simulink model "Missile_Plant_Trim_Analysis"  (R2021b)
settings: Solver=ode4  StartTime=0.0  StopTime=2  FixedStep=Step_Size  RelTol=1e-3
values from neighbouring files (symbols this model uses):
  D = 0.150    (= 0.15)    [Missile_Data.m]
  I_xx = 0.5 * Mass * ( D / 2 )^2    (= 0.084375)    [Missile_Data.m]
  I_yy = Mass * ( ( 1 / 12 ) * l^2 + ( 1 / 4 ) * ( D / 2 )^2 )    (= 6.5869975)    [Missile_Data.m]
  I_zz = I_yy    (= 6.5869975)    [Missile_Data.m]
  Mass = 30.0    (= 30)    [Missile_Data.m]
  S = ( pi / 4 ) * D^2    (= 0.0176714586764)    [Missile_Data.m]
  Tbl_CL_ALPHAT = [ -0.0988   -0.4859   -0.5870   -0.4802   -0.3334   -0.0210 ]    [Missile_Data.m]
  Tbl_CL_DEL_R = [ 5.2712    5.7640    6.1650    6.6234    7.1963    8.4110 ]    [Missile_Data.m]
  Tbl_CL_P = [ -17.9516  -19.6297  -20.9956  -22.5566  -24.5079  -28.6446 ]    [Missile_Data.m]
  Tbl_CM_0 = [ 0   -2.2250   -3.9280   -4.8580   -5.6940 ... (first row only)    [Missile_Data.m]
  Tbl_CM_DEL_P = [ -20.7182  -22.5631  -23.6059  -24.7632  -26.1269  -29.5646 ]    [Missile_Data.m]
  Tbl_CM_PHIT = [ 0   -0.0024   -0.0898   -0.2360   -0.3546 ... (first row only)    [Missile_Data.m]
  Tbl_CM_Q = [ -82.9643  -47.4409  -32.7732  -16.7304  -43.2010  -56.1499 ]    [Missile_Data.m]
  Tbl_CN_DEL_Y = [ -0.3616   -0.3938   -0.4120   -0.4322   -0.4560   -0.5160 ]    [Missile_Data.m]
  Tbl_CN_PHIT = [ 0    0.0040    0.0098    0.1116    0.3049 ... (first row only)    [Missile_Data.m]
  Tbl_CN_R = [ -82.9643  -47.4409  -32.7732  -16.7304  -43.2010  -56.1499 ]    [Missile_Data.m]
  Tbl_CX_0 = [ -0.3840   -0.3670   -0.3550   -0.3460   -0.3390   -0.3410 ]    [Missile_Data.m]
  Tbl_CX_ALPHAT = [ 0.0788    0.0752    0.0680    0.0573    0.0573    0.0573 ]    [Missile_Data.m]
  Tbl_CX_DEL_EFF = [ -16.8080  -17.8585  -18.9090  -19.9595  -20.4847  -23.1110 ]    [Missile_Data.m]
  Tbl_CY_DEL_Y = [ 5.3056    5.7754    6.0504    6.3484    6.6921    7.5745 ]    [Missile_Data.m]
  Tbl_CY_PHIT = [ 0    0.0070    0.0819    0.2313    0.2992 ... (first row only)    [Missile_Data.m]
  Tbl_CZ_0 = [ 0   -2.0680   -3.9700   -5.4250   -6.6810 ... (first row only)    [Missile_Data.m]
  Tbl_CZ_DEL_P = [ -5.3056   -5.7754   -6.0504   -6.3484   -6.6921   -7.5745 ]    [Missile_Data.m]
  Tbl_CZ_PHIT = [ 0    0.0089    0.1842    0.3041    0.2039 ... (first row only)    [Missile_Data.m]
  UNIT_GRAV = 9.81    [Sim_Parameters.m]
  windOn = 0    [Sim_Parameters.m]
  XCG = 0.809    [Missile_Data.m]
  XREF = 0.809    [Missile_Data.m]
undefined symbols (not defined in the file or in its folder): F, Light, MIL
libraries: aerolibwind2 x3, aerolibasang x3, sharedtransform x2, aerolibatmos2 x1, shared6dof x1, aerolibnav x1, sharedutil x1, simulink_extras x1
settings Model: Creator=Tiga  LastModifiedBy=Tiga
settings DataIOCC: SaveOutput=off  SaveTime=off

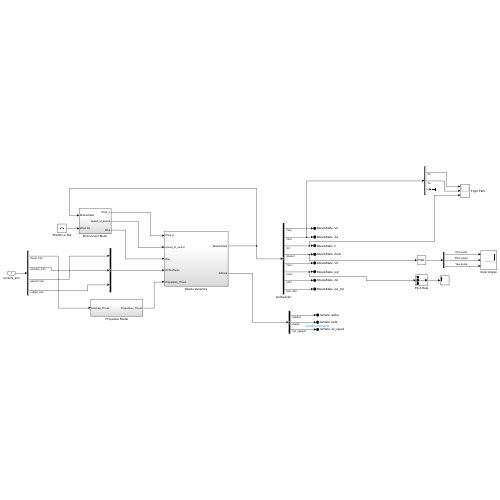
[thumbnail: Simulink's stored preview of the top-level diagram]
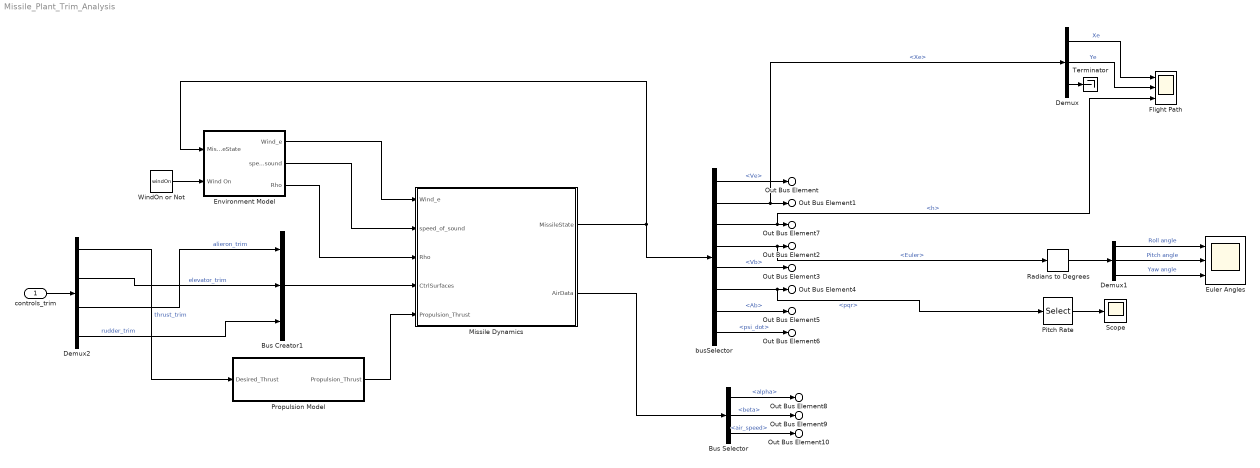
== system Missile_Plant_Trim_Analysis ==
  controls_trim : Inport
  Bus Creator1 : BusCreator  Inputs=3
  Bus Selector : BusSelector  OutputSignals=alpha,beta,air_speed
  Demux : Demux  Outputs=3
  Demux1 : Demux  Outputs=3
  Demux2 : Demux
  Environment Model : Subsystem
  Euler Angles : Scope  NumInputPorts=3
  Flight Path : Scope  NumInputPorts=3
  Missile Dynamics : Subsystem
  Pitch Rate : Selector  InputPortWidth=3  IndexOptions=Index vector (dialog)  Indices=[2]  OutputSizes=1
  Propulsion Model : Subsystem
  Radians to Degrees : simulink_extras/Transformations/Radians to Degrees
  Scope : Scope
  Terminator : Terminator
  WindOn or Not : Constant  Value=windOn
  busSelector : BusSelector  OutputSignals=Ve,Xe,h,Euler,Vb,pqr,Ab,psi_dot
  Out Bus Element : Outport  PortName=MissileState  Element=Ve
  Out Bus Element1 : Outport  PortName=MissileState  Element=Xe
  Out Bus Element2 : Outport  PortName=MissileState  Element=Euler
  Out Bus Element3 : Outport  PortName=MissileState  Element=Vb
  Out Bus Element4 : Outport  PortName=MissileState  Element=pqr
  Out Bus Element5 : Outport  PortName=MissileState  Element=Ab
  Out Bus Element6 : Outport  PortName=MissileState  Element=psi_dot
  Out Bus Element7 : Outport  PortName=MissileState  Element=h
  Out Bus Element8 : Outport  Port=2  PortName=AirData  Element=alpha
  Out Bus Element9 : Outport  Port=2  PortName=AirData  Element=beta
  Out Bus Element10 : Outport  Port=2  PortName=AirData  Element=air_speed
  wires:
  busSelector/8 -> Out Bus Element6/1  "<psi_dot>"
  busSelector/7 -> Out Bus Element5/1  "<Ab>"
  busSelector/6 -> Pitch Rate/1, Out Bus Element4/1  "<pqr>"
  busSelector/5 -> Out Bus Element3/1  "<Vb>"
  busSelector/4 -> Radians to Degrees/1, Out Bus Element2/1  "<Euler>"
  busSelector/2 -> Out Bus Element1/1, Demux/1  "<Xe>"
  busSelector/1 -> Out Bus Element/1  "<Ve>"
  Missile Dynamics/1(MissileState) -> busSelector/1, Environment Model/1(MissileState)
  Environment Model/3(Rho) -> Missile Dynamics/3(Rho)
  WindOn or Not/1 -> Environment Model/2(Wind On)
  Environment Model/1(Wind_e) -> Missile Dynamics/1(Wind_e)
  Propulsion Model/1(Propulsion_Thrust) -> Missile Dynamics/5(Propulsion_Thrust)
  Environment Model/2(speed_of_sound) -> Missile Dynamics/2(speed_of_sound)
  busSelector/3 -> Flight Path/3, Out Bus Element7/1  "<h>"
  Radians to Degrees/1 -> Demux1/1
  Demux1/2 -> Euler Angles/2  "Pitch angle"
  Demux1/3 -> Euler Angles/3  "Yaw angle"
  Demux1/1 -> Euler Angles/1  "Roll angle"
  Pitch Rate/1 -> Scope/1
  Demux/1 -> Flight Path/1  "Xe"
  Demux/2 -> Flight Path/2  "Ye"
  Demux/3 -> Terminator/1
  controls_trim/1 -> Demux2/1
  Demux2/1 -> Propulsion Model/1(Desired_Thrust)  "thrust_trim"
  Demux2/3 -> Bus Creator1/1  "alieron_trim"
  Demux2/2 -> Bus Creator1/2  "elevator_trim"
  Demux2/4 -> Bus Creator1/3  "rudder_trim"
  Bus Creator1/1 -> Missile Dynamics/4(CtrlSurfaces)
  Missile Dynamics/2(AirData) -> Bus Selector/1
  Bus Selector/1 -> Out Bus Element8/1  "<alpha>"
  Bus Selector/2 -> Out Bus Element9/1  "<beta>"
  Bus Selector/3 -> Out Bus Element10/1  "<air_speed>"

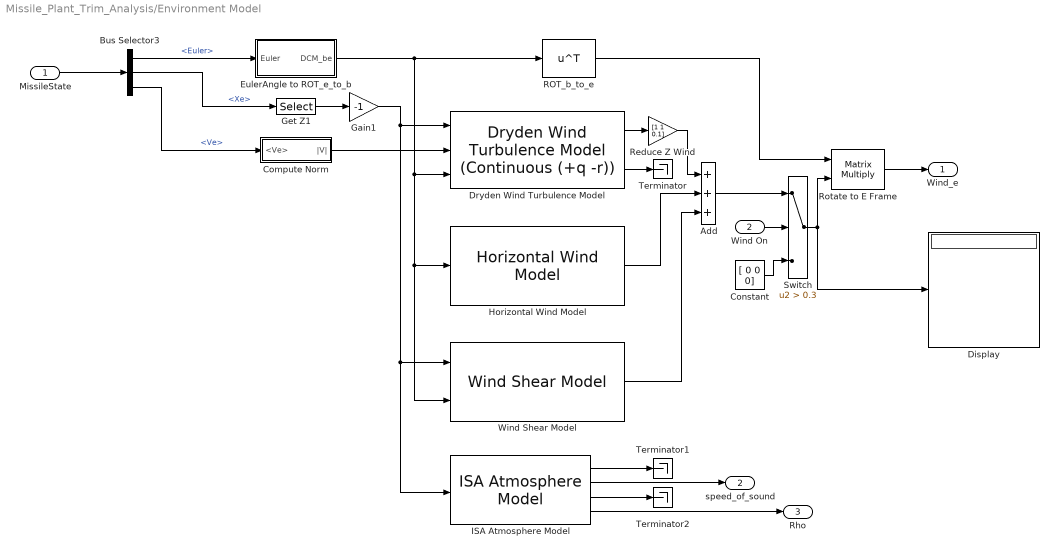
== system Missile_Plant_Trim_Analysis/Environment Model ==
  MissileState : Inport
  Wind On : Inport  Port=2
  Add : Sum  Inputs=3
  Bus Selector3 : BusSelector  OutputSignals=Euler,Xe,Ve
  Compute Norm : Subsystem
  Constant : Constant  Value=[ 0 0 0]
      settings: AttributesFormatString=%<Value>
  Display : Display
  Dryden Wind Turbulence Model : aerolibwind2/Dryden Wind Turbulence Model  (Continuous (+q -r))  units=Metric (MKS)  spec=MIL-F-8785C  model=Continuous Dryden (+q -r)  W20=12  Wdeg=180  TurbProb=10^-2 - Light  L_high=533.4  Wingspan=l  ts=0.01  Seed=[23341 23342 23343 23344]  T_on=on
  EulerAngle to ROT_e_to_b : Subsystem
  Gain1 : Gain  Gain=-1
      settings: AttributesFormatString=Z to Alt
  Get Z1 : Selector  InputPortWidth=3  IndexOptions=Index vector (dialog)  Indices=[3]  OutputSizes=[(-2)]
  "Horizontal Wind Model " : aerolibwind2/Horizontal Wind Model  units=Metric (MKS)  Vw_source=Internal  Vwind=12  W_source=Internal  Wdeg=90
      settings: SourceProductBaseCode=AE
  ISA Atmosphere Model : aerolibatmos2/ISA Atmosphere Model  custom=off  g=9.80665  gamma=1.4  R=287.0531  L=0.0065  h_trop=11000  h_strat=20000  rho0=1.225  P0=101325  T0=288.15  h0=0
  ROT_b_to_e : Math  Operator=transpose  SignedPower=on  SaturateOnIntegerOverflow=on
  Reduce Z Wind : Gain  Gain=[1 1 0.1]
      settings: AttributesFormatString=%<Gain>
  Rotate to E Frame : Product  Multiplication=Matrix(*)
  Switch : Switch  Criteria=u2 > Threshold  Threshold=0.3
  Terminator : Terminator
  Terminator1 : Terminator
  Terminator2 : Terminator
  Wind Shear Model : aerolibwind2/Wind Shear Model  units=Metric (MKS)  phase=Category C - Terminal Flight Phase  W_20=15  Wdeg=0
  Wind_e : Outport  Unit=m/s  VectorParamsAs1DForOutWhenUnconnected=off
  speed_of_sound : Outport  Port=2  Unit=m/s  VectorParamsAs1DForOutWhenUnconnected=off
  Rho : Outport  Port=3  Unit=kg/m^3  VectorParamsAs1DForOutWhenUnconnected=off
  wires:
  Compute Norm/1(|V|) -> Dryden Wind Turbulence Model/2
  Bus Selector3/3 -> Compute Norm/1(<Ve>)  "<Ve>"
  EulerAngle to ROT_e_to_b/1(DCM_be) -> ROT_b_to_e/1, Dryden Wind Turbulence Model/3, "Horizontal Wind Model "/1, Wind Shear Model/2
  Bus Selector3/1 -> EulerAngle to ROT_e_to_b/1(Euler)  "<Euler>"
  ISA Atmosphere Model/3 -> Terminator2/1
  ISA Atmosphere Model/1 -> Terminator1/1
  ISA Atmosphere Model/2 -> speed_of_sound/1
  ISA Atmosphere Model/4 -> Rho/1
  Wind Shear Model/1 -> Add/3
  Wind On/1 -> Switch/2
  Add/1 -> Switch/1
  Reduce Z Wind/1 -> Add/1
  "Horizontal Wind Model "/1 -> Add/2
  Gain1/1 -> Dryden Wind Turbulence Model/1, Wind Shear Model/1, ISA Atmosphere Model/1
  MissileState/1 -> Bus Selector3/1
  Dryden Wind Turbulence Model/1 -> Reduce Z Wind/1
  Switch/1 -> Display/1, Rotate to E Frame/2
  Rotate to E Frame/1 -> Wind_e/1
  ROT_b_to_e/1 -> Rotate to E Frame/1
  Get Z1/1 -> Gain1/1
  Constant/1 -> Switch/3
  Dryden Wind Turbulence Model/2 -> Terminator/1
  Bus Selector3/2 -> Get Z1/1  "<Xe>"

== system Missile_Plant_Trim_Analysis/Missile Dynamics ==
  Wind_e : Inport
  speed_of_sound : Inport  Port=2
  Rho : Inport  Port=3
  CtrlSurfaces : Inport  Port=4
  Propulsion_Thrust : Inport  Port=5
  6DOF Nonlinear Equations of Motion : Subsystem
  Aerodynamic Forces and Moments : Subsystem
  Total Force and Moment : Subsystem
  MissileState : Outport
  AirData : Outport  Port=2
  wires:
  CtrlSurfaces/1 -> Aerodynamic Forces and Moments/5(CtrlSurfaces)
  Rho/1 -> Aerodynamic Forces and Moments/4(Rho)
  speed_of_sound/1 -> Aerodynamic Forces and Moments/3(speed_of_sound)
  Wind_e/1 -> Aerodynamic Forces and Moments/1(Wind_e)
  6DOF Nonlinear Equations of Motion/1(MissileState) -> Aerodynamic Forces and Moments/2(MissileState), MissileState/1, Total Force and Moment/3(MissileState)
  Propulsion_Thrust/1 -> Total Force and Moment/2(Propulsion_Thrust)
  Aerodynamic Forces and Moments/1(Fm_b) -> Total Force and Moment/1(Aero-Force-Moment)
  Total Force and Moment/1(Total_Force_Moment) -> 6DOF Nonlinear Equations of Motion/1(FM_b)
  Aerodynamic Forces and Moments/2(AirData) -> AirData/1

== system Missile_Plant_Trim_Analysis/Propulsion Model ==
  note: F_Tx
  Desired_Thrust : Inport
  F_Ty : Constant  Value=0
  F_Tz : Constant  Value=0
  L_T : Constant  Value=0
  M_T : Constant  Value=0
  Mux : Mux  Inputs=3
  Mux1 : Mux  Inputs=3
  Mux2 : Mux  Inputs=2
  N_T : Constant  Value=0
  Propulsion_Thrust : Outport
  wires:
  N_T/1 -> Mux1/3
  M_T/1 -> Mux1/2
  L_T/1 -> Mux1/1
  F_Tz/1 -> Mux/3
  F_Ty/1 -> Mux/2
  Desired_Thrust/1 -> Mux/1
  Mux2/1 -> Propulsion_Thrust/1
  Mux1/1 -> Mux2/2
  Mux/1 -> Mux2/1

== system Missile_Plant_Trim_Analysis/Environment Model/Compute Norm ==
  <Ve> : Inport
  Dot Product : DotProduct  InputSameDT=on  OutDataTypeStr=Inherit: Inherit via internal rule
  Sqrt : Sqrt  SaturateOnIntegerOverflow=on
  Zero Bound : Saturate  UpperLimit=inf  LowerLimit=0.001
      settings: AttributesFormatString="[%<LowerLimit>  %<UpperLimit>]"
  |V| : Outport
  wires:
  Zero Bound/1 -> Sqrt/1
  Dot Product/1 -> Zero Bound/1
  Sqrt/1 -> |V|/1
  <Ve>/1 -> Dot Product/1, Dot Product/2

== system Missile_Plant_Trim_Analysis/Environment Model/EulerAngle to ROT_e_to_b ==
  Euler : Inport
  Rotation Angles to Direction Cosine Matrix : sharedtransform/Rotation Angles to Direction Cosine Matrix  rotationOrder=ZYX  aMode=aMode
      settings: SourceProductBaseCode=AE,PW,DR,MT,UV,VE
  Selector : Selector  InputPortWidth=3  IndexOptions=Index vector (dialog)  Indices=[3 2 1]  OutputSizes=1
  DCM_be : Outport
  wires:
  Euler/1 -> Selector/1
  Selector/1 -> Rotation Angles to Direction Cosine Matrix/1  "3 (rad)"
  Rotation Angles to Direction Cosine Matrix/1 -> DCM_be/1

== system Missile_Plant_Trim_Analysis/Missile Dynamics/6DOF Nonlinear Equations of Motion ==
  FM_b : Inport
  6DOF (Euler Angles) : shared6dof/6DOF (Euler Angles)  units=Metric (MKS)  mtype=Fixed  rep=Euler Angles  xme_0=Init_Pos  Vm_0=Init_Vel  eul_0=[ 0.0, 0.0, 0.0 ]  pm_0=Init_Rate  mass_0=Mass  mass_e=0.5  mass_f=2.0  inertia=eye(3).*[I_xx;I_yy;I_zz]  inertia_e=eye(3)  inertia_f=2*eye(3)  k_quat=1.0  vre_flag=on  abi_flag=off  aMode=aMode  xme_statename=''  Vm_statename=''  eul_statename=''  quat_statename=''  pm_statename=''  mass_statename=''
      settings: SourceProductBaseCode=AE
  Bus Creator : BusCreator  Inputs=9
  Compute psi_dot : Subsystem
  Constant : Constant  Value=[0 0 0]
      settings: AttributesFormatString=%<Value>
  Demux2 : Demux  Outputs=2
  Three-axis Accelerometer : aerolibnav/Three-axis Accelerometer  units=Metric (MKS)  acc=[0 0 0]  gtype=off  dtype_a=off  w_a=190  z_a=0.707  a_sf_cc=[1 0 0; 0 1 0; 0 0 1]  a_bias=[0 0 0]  a_Ts=0  a_rand=off  a_seeds=[23093 23094 23095]  a_pow=[0.001 0.001 0.001]  a_sat="[-inf  -inf  -inf  inf inf inf]"
      settings: SourceProductBaseCode=AE
  Z_to_Altitude : Subsystem
  MissileState : Outport
  wires:
  Bus Creator/1 -> MissileState/1
  Three-axis Accelerometer/1 -> Bus Creator/8  "Ab"
  6DOF (Euler Angles)/2 -> Z_to_Altitude/1(Xe), Bus Creator/2  "Xe"
  Demux2/1 -> 6DOF (Euler Angles)/1
  6DOF (Euler Angles)/6 -> Three-axis Accelerometer/2, Bus Creator/7, Compute psi_dot/2(G)  "pqr"
  Demux2/2 -> 6DOF (Euler Angles)/2
  6DOF (Euler Angles)/1 -> Bus Creator/1  "Ve"
  6DOF (Euler Angles)/7 -> Three-axis Accelerometer/3
  6DOF (Euler Angles)/5 -> Bus Creator/6  "Vb"
  Constant/1 -> Three-axis Accelerometer/4
  6DOF (Euler Angles)/3 -> Compute psi_dot/1(Euler), Bus Creator/4  "Euler"
  FM_b/1 -> Demux2/1
  Compute psi_dot/1(psi_dot) -> Bus Creator/9  "psi_dot"
  6DOF (Euler Angles)/8 -> Three-axis Accelerometer/1
  6DOF (Euler Angles)/4 -> Bus Creator/5  "DCM_be"
  Z_to_Altitude/1(h) -> Bus Creator/3  "h"

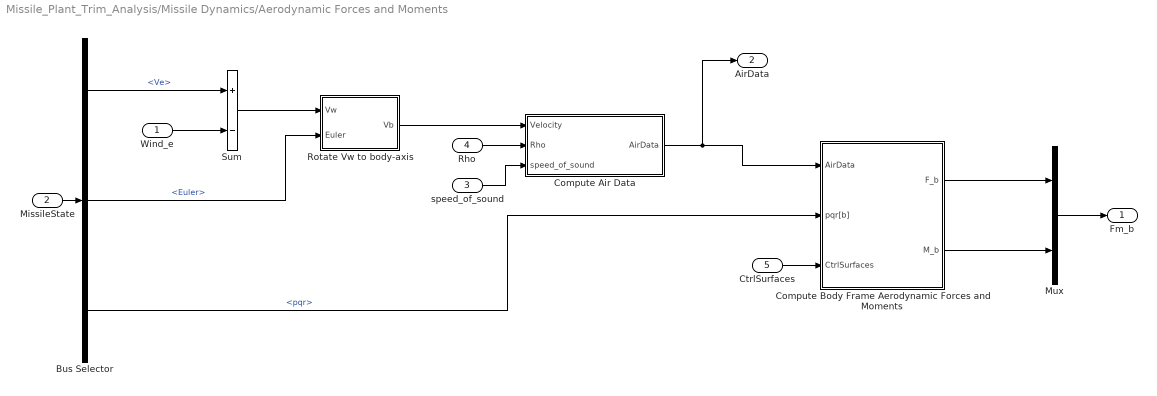
== system Missile_Plant_Trim_Analysis/Missile Dynamics/Aerodynamic Forces and Moments ==
  Wind_e : Inport
  MissileState : Inport  Port=2
  speed_of_sound : Inport  Port=3  Unit=m/s
  Rho : Inport  Port=4  Unit=kg/m^3
  CtrlSurfaces : Inport  Port=5
  Bus Selector : BusSelector  OutputSignals=Ve,Euler,pqr
  Compute Air Data : Subsystem
  Compute Body Frame Aerodynamic Forces and Moments : Subsystem
  Mux : Mux  Inputs=2
  Rotate Vw to body-axis : Subsystem
  Sum : Sum  Inputs=+-
  Fm_b : Outport
  AirData : Outport  Port=2
  wires:
  Compute Body Frame Aerodynamic Forces and Moments/1(F_b) -> Mux/1
  Compute Body Frame Aerodynamic Forces and Moments/2(M_b) -> Mux/2
  Mux/1 -> Fm_b/1
  CtrlSurfaces/1 -> Compute Body Frame Aerodynamic Forces and Moments/3(CtrlSurfaces)
  Compute Air Data/1(AirData) -> AirData/1, Compute Body Frame Aerodynamic Forces and Moments/1(AirData)
  speed_of_sound/1 -> Compute Air Data/3(speed_of_sound)
  Rho/1 -> Compute Air Data/2(Rho)
  Rotate Vw to body-axis/1(Vb) -> Compute Air Data/1(Velocity)
  Bus Selector/2 -> Rotate Vw to body-axis/2(Euler)  "<Euler>"
  Bus Selector/3 -> Compute Body Frame Aerodynamic Forces and Moments/2(pqr[b])  "<pqr>"
  MissileState/1 -> Bus Selector/1
  Wind_e/1 -> Sum/2
  Sum/1 -> Rotate Vw to body-axis/1(Vw)
  Bus Selector/1 -> Sum/1  "<Ve>"

== system Missile_Plant_Trim_Analysis/Missile Dynamics/Total Force and Moment ==
  Aero-Force-Moment : Inport
  Propulsion_Thrust : Inport  Port=2
  MissileState : Inport  Port=3
  Demux : Demux  Outputs=2
  Demux1 : Demux  Outputs=2
  Gravity : Subsystem
  Gravity's effect on moment : Constant  Value=0
  Mux : Mux  Inputs=2
  Total Force : Sum  Inputs=+++
  Total Moment : Sum  Inputs=+++
  Total_Force_Moment : Outport
  wires:
  Aero-Force-Moment/1 -> Demux/1
  Propulsion_Thrust/1 -> Demux1/1
  Demux/1 -> Total Force/1  "Aero-F"
  Demux1/1 -> Total Force/2  "Prop-F"
  MissileState/1 -> Gravity/1(MissileState)
  Gravity/1(Gravitational Force) -> Total Force/3  "Gravity-F"
  Demux/2 -> Total Moment/1  "Aero-M"
  Demux1/2 -> Total Moment/2  "Prop-M"
  Gravity's effect on moment/1 -> Total Moment/3
  Total Force/1 -> Mux/1
  Total Moment/1 -> Mux/2
  Mux/1 -> Total_Force_Moment/1

== system Missile_Plant_Trim_Analysis/Missile Dynamics/6DOF Nonlinear Equations of Motion/Compute psi_dot ==
  Euler : Inport
  G : Inport  Port=2
  Mux1 : Mux  Inputs=2
  psidot : Fcn  Expr=(u[5]*sin(u[1])+u[6]*cos(u[1]))/cos(u[2])
  psi_dot : Outport  Unit=rad/S  VectorParamsAs1DForOutWhenUnconnected=off
  wires:
  Euler/1 -> Mux1/1
  Mux1/1 -> psidot/1
  psidot/1 -> psi_dot/1  "psi_dot"
  G/1 -> Mux1/2

== system Missile_Plant_Trim_Analysis/Missile Dynamics/6DOF Nonlinear Equations of Motion/Z_to_Altitude ==
  Xe : Inport
  Gain : Gain  Gain=-1
  Selector : Selector  InputPortWidth=3  IndexOptions=Index vector (dialog)  Indices=[3]  OutputSizes=1
  h : Outport
  wires:
  Xe/1 -> Selector/1
  Selector/1 -> Gain/1
  Gain/1 -> h/1

== system Missile_Plant_Trim_Analysis/Missile Dynamics/Aerodynamic Forces and Moments/Compute Air Data ==
  Velocity : Inport
  Rho : Inport  Port=2  Unit=kg/m^3
  speed_of_sound : Inport  Port=3  Unit=m/s
  Bus Creator : BusCreator  Inputs=5
  Dynamic Pressure : aerolibasang/Dynamic Pressure
  "Incidence, Sideslip, & Airspeed" : aerolibasang/Incidence, Sideslip, & Airspeed
  Mach Number : aerolibasang/Mach Number
      settings: SourceProductBaseCode=AE
  AirData : Outport
  wires:
  "Incidence, Sideslip, & Airspeed"/3 -> Bus Creator/3  "air_speed"
  Bus Creator/1 -> AirData/1
  speed_of_sound/1 -> Mach Number/2
  "Incidence, Sideslip, & Airspeed"/2 -> Bus Creator/2  "beta"
  Dynamic Pressure/1 -> Bus Creator/4  "dynamic_pressure"
  "Incidence, Sideslip, & Airspeed"/1 -> Bus Creator/1  "alpha"
  Rho/1 -> Dynamic Pressure/2
  Mach Number/1 -> Bus Creator/5  "mach"
  Velocity/1 -> Dynamic Pressure/1, Mach Number/1, "Incidence, Sideslip, & Airspeed"/1

== system Missile_Plant_Trim_Analysis/Missile Dynamics/Aerodynamic Forces and Moments/Compute Body Frame Aerodynamic Forces and Moments ==
  AirData : Inport
  pqr[b] : Inport  Port=2
  CtrlSurfaces : Inport  Port=3
  Bus Selector : BusSelector  OutputSignals=dynamic_pressure
  Compute Aeroballistics Frame Aerodynamics Coefficients : Subsystem
  Compute Body Frame Aerodynamic Forces and Moments : Subsystem
  Convert AeroCoeffs_a to AeroCoeffs_b : Subsystem
  Display : Display
  F_b : Outport
  M_b : Outport  Port=2
  wires:
  Convert AeroCoeffs_a to AeroCoeffs_b/2(Aero-M-Coeffs_b) -> Compute Body Frame Aerodynamic Forces and Moments/3(Aero-M-Coeffs_b)
  Compute Aeroballistics Frame Aerodynamics Coefficients/2(Aero-M-Coeffs_a) -> Convert AeroCoeffs_a to AeroCoeffs_b/2(Aero-M-Coeffs_a)
  Compute Aeroballistics Frame Aerodynamics Coefficients/3(ROT_b_to_a) -> Convert AeroCoeffs_a to AeroCoeffs_b/3(ROT_b_to_a)
  Bus Selector/1 -> Compute Body Frame Aerodynamic Forces and Moments/1(dynamic_pressure)  "<dynamic_pressure>"
  Compute Body Frame Aerodynamic Forces and Moments/2(M_b) -> M_b/1
  Convert AeroCoeffs_a to AeroCoeffs_b/1(Aero-F-Coeffs_b) -> Compute Body Frame Aerodynamic Forces and Moments/2(Aero-F-Coeffs_b)
  Compute Body Frame Aerodynamic Forces and Moments/1(F_b) -> F_b/1
  Compute Aeroballistics Frame Aerodynamics Coefficients/1(Aero-F-Coeffs_a) -> Convert AeroCoeffs_a to AeroCoeffs_b/1(Aero-F-Coeffs_a)
  pqr[b]/1 -> Compute Aeroballistics Frame Aerodynamics Coefficients/2(pqr[b])
  CtrlSurfaces/1 -> Compute Aeroballistics Frame Aerodynamics Coefficients/3(CtrlSurfaces)
  AirData/1 -> Display/1, Compute Aeroballistics Frame Aerodynamics Coefficients/1(AirData), Bus Selector/1

== system Missile_Plant_Trim_Analysis/Missile Dynamics/Aerodynamic Forces and Moments/Rotate Vw to body-axis ==
  Vw : Inport
  Euler : Inport  Port=2
  EulerAngle to ROT_e_to_b : Subsystem
  RL2B * Vw : Product  Multiplication=Matrix(*)  InputSameDT=on  SaturateOnIntegerOverflow=on  OutDataTypeStr=Inherit: Same as first input
  Vb : Outport  Unit=m/s  VectorParamsAs1DForOutWhenUnconnected=off
  wires:
  EulerAngle to ROT_e_to_b/1(DCM_be) -> RL2B * Vw/1
  Euler/1 -> EulerAngle to ROT_e_to_b/1(Euler)
  Vw/1 -> RL2B * Vw/2
  RL2B * Vw/1 -> Vb/1

== system Missile_Plant_Trim_Analysis/Missile Dynamics/Total Force and Moment/Gravity ==
  MissileState : Inport
  Bus Selector : BusSelector  OutputSignals=DCM_be
  Constant : Constant  Value=Mass
  Constant1 : Constant  Value=0
  Matrix Multiply : Product  Multiplication=Matrix(*)
  Mux : Mux  Inputs=3
  UNIT_GRAV : Gain  Gain=UNIT_GRAV
  Gravitational Force : Outport
  wires:
  UNIT_GRAV/1 -> Mux/3
  Constant/1 -> UNIT_GRAV/1
  Constant1/1 -> Mux/2, Mux/1
  MissileState/1 -> Bus Selector/1
  Bus Selector/1 -> Matrix Multiply/1  "<DCM_be>"
  Mux/1 -> Matrix Multiply/2
  Matrix Multiply/1 -> Gravitational Force/1

== system Missile_Plant_Trim_Analysis/Missile Dynamics/Aerodynamic Forces and Moments/Compute Body Frame Aerodynamic Forces and Moments/Compute Aeroballistics Frame Aerodynamics Coefficients ==
  AirData : Inport
  pqr[b] : Inport  Port=2
  CtrlSurfaces : Inport  Port=3
  Calculate Coefficient Parameters : Subsystem
  Compute Aero-F-Coeffs_a : Subsystem
  Compute Aero-M-Coeffs_a : Subsystem
  Mach_Number Index Search : PreLookup  BreakpointsData=Tbl_MACH  OutputSelection=Index and fraction as bus  ExtrapMethod=Linear
  alpha_T Index Search : PreLookup  BreakpointsData=Tbl_ALPHAT  OutputSelection=Index and fraction as bus  BeginIndexSearchUsingPreviousIndexResult=on  ExtrapMethod=Linear
  Aero-F-Coeffs_a : Outport
  Aero-M-Coeffs_a : Outport  Port=2
  ROT_b_to_a : Outport  Port=3
  wires:
  Compute Aero-M-Coeffs_a/1(Aero-M-Coeffs_a) -> Aero-M-Coeffs_a/1
  Calculate Coefficient Parameters/9(pqr[a]) -> Compute Aero-M-Coeffs_a/8(pqr[a])
  Calculate Coefficient Parameters/8(geo_param) -> Compute Aero-M-Coeffs_a/7(geo_param)
  Calculate Coefficient Parameters/7(D/2V) -> Compute Aero-M-Coeffs_a/6(D/2V)
  Compute Aero-F-Coeffs_a/1(Aero-F-Coeffs_a) -> Aero-F-Coeffs_a/1, Compute Aero-M-Coeffs_a/9(Aero-F-Coeffs_a)
  Calculate Coefficient Parameters/6(roll_angle_T) -> Compute Aero-M-Coeffs_a/3(roll_angle_T), Compute Aero-F-Coeffs_a/4(roll_angle_T)
  Calculate Coefficient Parameters/5(CtrlSurfaces[a]) -> Compute Aero-M-Coeffs_a/5(CtrlSurfaces[a]), Compute Aero-F-Coeffs_a/6(CtrlSurfaces[a])
  Calculate Coefficient Parameters/4(dEFF) -> Compute Aero-F-Coeffs_a/5(dEFF)
  Mach_Number Index Search/1 -> Compute Aero-F-Coeffs_a/2(Mach_Number_index), Compute Aero-M-Coeffs_a/2(Mach_Number_index)
  alpha_T Index Search/1 -> Compute Aero-F-Coeffs_a/1(alpha_T_index), Compute Aero-M-Coeffs_a/1(alpha_T_index)
  Calculate Coefficient Parameters/3(Mach_Number) -> Mach_Number Index Search/1
  Calculate Coefficient Parameters/2(alpha_T) -> Compute Aero-F-Coeffs_a/3(alpha_T), Compute Aero-M-Coeffs_a/4(alpha_T), alpha_T Index Search/1
  Calculate Coefficient Parameters/1(ROT_b_to_a) -> ROT_b_to_a/1
  AirData/1 -> Calculate Coefficient Parameters/1(AirData)
  pqr[b]/1 -> Calculate Coefficient Parameters/2(pqr[b])
  CtrlSurfaces/1 -> Calculate Coefficient Parameters/3(CtrlSurfaces[b])

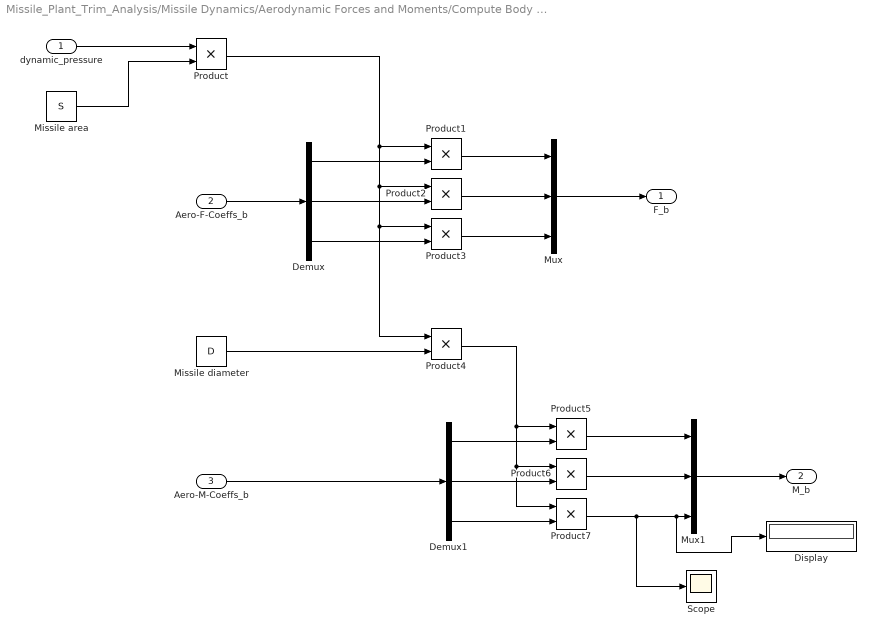
== system Missile_Plant_Trim_Analysis/Missile Dynamics/Aerodynamic Forces and Moments/Compute Body Frame Aerodynamic Forces and Moments/Compute Body Frame Aerodynamic Forces and Moments ==
  dynamic_pressure : Inport
  Aero-F-Coeffs_b : Inport  Port=2
  Aero-M-Coeffs_b : Inport  Port=3
  Demux : Demux  Outputs=3
  Demux1 : Demux  Outputs=3
  Display : Display
  Missile area : Constant  Value=S
  "Missile diameter " : Constant  Value=D
  Mux : Mux  Inputs=3
  Mux1 : Mux  Inputs=3
  Product{,1..7} (8 alike) : Product
  Scope : Scope
  F_b : Outport
  M_b : Outport  Port=2
  wires:
  Product7/1 -> Scope/1, Display/1, Mux1/3
  Demux1/3 -> Product7/2
  Product6/1 -> Mux1/2
  Demux1/2 -> Product6/2
  Product5/1 -> Mux1/1
  Demux1/1 -> Product5/2
  Product4/1 -> Product5/1, Product7/1, Product6/1
  "Missile diameter "/1 -> Product4/2
  Mux1/1 -> M_b/1
  Product3/1 -> Mux/3
  Demux/3 -> Product3/2
  Product2/1 -> Mux/2
  Demux/2 -> Product2/2
  Product1/1 -> Mux/1
  Demux/1 -> Product1/2
  Product/1 -> Product1/1, Product2/1, Product3/1, Product4/1
  Missile area/1 -> Product/2
  dynamic_pressure/1 -> Product/1
  Mux/1 -> F_b/1
  Aero-M-Coeffs_b/1 -> Demux1/1
  Aero-F-Coeffs_b/1 -> Demux/1

== system Missile_Plant_Trim_Analysis/Missile Dynamics/Aerodynamic Forces and Moments/Compute Body Frame Aerodynamic Forces and Moments/Convert AeroCoeffs_a to AeroCoeffs_b ==
  Aero-F-Coeffs_a : Inport
  Aero-M-Coeffs_a : Inport  Port=2
  ROT_b_to_a : Inport  Port=3
  Bus to Vector : BusToVector
  Bus to Vector1 : BusToVector
  Matrix Multiply : Product  Multiplication=Matrix(*)
  Matrix Multiply1 : Product  Multiplication=Matrix(*)
  ROT_a_to_b : Math  Operator=transpose  SaturateOnIntegerOverflow=on
  Reshape : Reshape  OutputDimensionality=Column vector (2-D)
  Reshape1 : Reshape  OutputDimensionality=Column vector (2-D)
  Aero-F-Coeffs_b : Outport
  Aero-M-Coeffs_b : Outport  Port=2
  wires:
  Bus to Vector1/1 -> Reshape1/1
  Aero-M-Coeffs_a/1 -> Bus to Vector1/1
  Bus to Vector/1 -> Reshape/1
  Aero-F-Coeffs_a/1 -> Bus to Vector/1
  Reshape1/1 -> Matrix Multiply1/2
  Reshape/1 -> Matrix Multiply/2
  ROT_a_to_b/1 -> Matrix Multiply1/1, Matrix Multiply/1
  Matrix Multiply1/1 -> Aero-M-Coeffs_b/1
  Matrix Multiply/1 -> Aero-F-Coeffs_b/1
  ROT_b_to_a/1 -> ROT_a_to_b/1

== system Missile_Plant_Trim_Analysis/Missile Dynamics/Aerodynamic Forces and Moments/Rotate Vw to body-axis/EulerAngle to ROT_e_to_b ==
  Euler : Inport
  Rotation Angles to Direction Cosine Matrix : sharedtransform/Rotation Angles to Direction Cosine Matrix  rotationOrder=ZYX  aMode=aMode
      settings: SourceProductBaseCode=AE,PW,DR,MT,UV,VE
  Selector : Selector  InputPortWidth=3  IndexOptions=Index vector (dialog)  Indices=[3 2 1]  OutputSizes=1
  DCM_be : Outport
  wires:
  Euler/1 -> Selector/1
  Selector/1 -> Rotation Angles to Direction Cosine Matrix/1  "3 (rad)"
  Rotation Angles to Direction Cosine Matrix/1 -> DCM_be/1

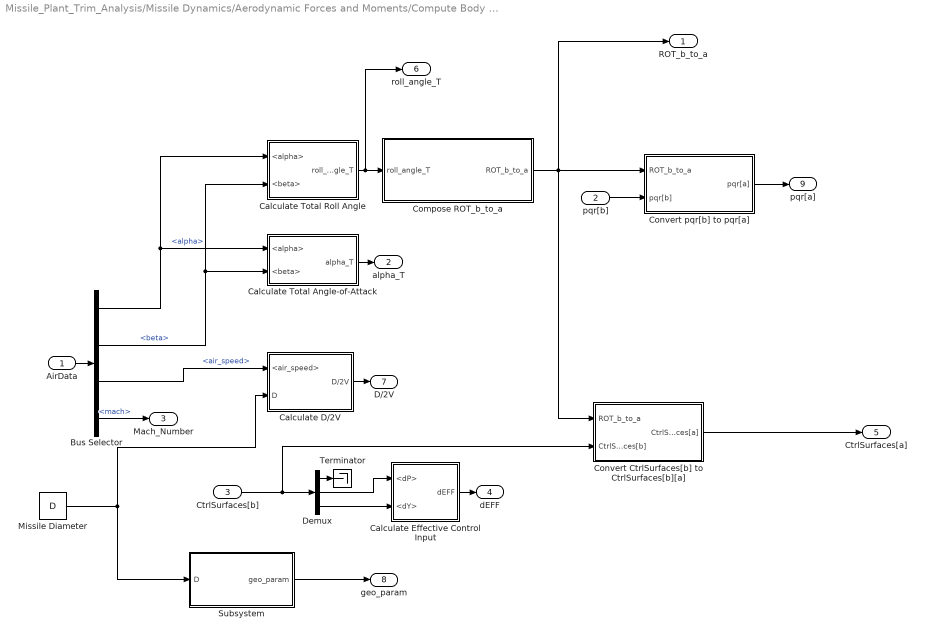
== system Missile_Plant_Trim_Analysis/Missile Dynamics/Aerodynamic Forces and Moments/Compute Body Frame Aerodynamic Forces and Moments/Compute Aeroballistics Frame Aerodynamics Coefficients/Calculate Coefficient Parameters ==
  AirData : Inport
  pqr[b] : Inport  Port=2
  CtrlSurfaces[b] : Inport  Port=3
  Bus Selector : BusSelector  OutputSignals=alpha,beta,air_speed,mach
  Calculate D/2V : Subsystem
  Calculate Effective Control Input : Subsystem
  Calculate Total Angle-of-Attack : Subsystem
  Calculate Total Roll Angle : Subsystem
  Compose ROT_b_to_a : Subsystem
  Convert CtrlSurfaces[b] to CtrlSurfaces[b][a] : Subsystem
  Convert pqr[b] to pqr[a] : Subsystem
  Demux : Demux  Outputs=3
  Missile Diameter : Constant  Value=D
  Subsystem : Subsystem
  Terminator : Terminator
  ROT_b_to_a : Outport
  alpha_T : Outport  Port=2
  Mach_Number : Outport  Port=3
  dEFF : Outport  Port=4
  CtrlSurfaces[a] : Outport  Port=5
  roll_angle_T : Outport  Port=6
  D/2V : Outport  Port=7
  geo_param : Outport  Port=8
  pqr[a] : Outport  Port=9
  wires:
  Subsystem/1(geo_param) -> geo_param/1
  Missile Diameter/1 -> Calculate D/2V/2(D), Subsystem/1(D)
  Bus Selector/4 -> Mach_Number/1  "<mach>"
  Bus Selector/3 -> Calculate D/2V/1(<air_speed>)  "<air_speed>"
  Bus Selector/2 -> Calculate Total Angle-of-Attack/2(<beta>), Calculate Total Roll Angle/2(<beta>)  "<beta>"
  Bus Selector/1 -> Calculate Total Angle-of-Attack/1(<alpha>), Calculate Total Roll Angle/1(<alpha>)  "<alpha>"
  AirData/1 -> Bus Selector/1
  Convert CtrlSurfaces[b] to CtrlSurfaces[b][a]/1(CtrlSurfaces[a]) -> CtrlSurfaces[a]/1
  Convert pqr[b] to pqr[a]/1(pqr[a]) -> pqr[a]/1
  Calculate Total Angle-of-Attack/1(alpha_T) -> alpha_T/1
  Calculate Effective Control Input/1(dEFF) -> dEFF/1
  CtrlSurfaces[b]/1 -> Convert CtrlSurfaces[b] to CtrlSurfaces[b][a]/2(CtrlSurfaces[b]), Demux/1
  Calculate Total Roll Angle/1(roll_angle_T) -> roll_angle_T/1, Compose ROT_b_to_a/1(roll_angle_T)
  Calculate D/2V/1(D/2V) -> D/2V/1
  pqr[b]/1 -> Convert pqr[b] to pqr[a]/2(pqr[b])
  Compose ROT_b_to_a/1(ROT_b_to_a) -> Convert pqr[b] to pqr[a]/1(ROT_b_to_a), Convert CtrlSurfaces[b] to CtrlSurfaces[b][a]/1(ROT_b_to_a), ROT_b_to_a/1
  Demux/1 -> Terminator/1
  Demux/2 -> Calculate Effective Control Input/1(<dP>)
  Demux/3 -> Calculate Effective Control Input/2(<dY>)

== system Missile_Plant_Trim_Analysis/Missile Dynamics/Aerodynamic Forces and Moments/Compute Body Frame Aerodynamic Forces and Moments/Compute Aeroballistics Frame Aerodynamics Coefficients/Compute Aero-F-Coeffs_a ==
  alpha_T_index : Inport
  Mach_Number_index : Inport  Port=2
  alpha_T : Inport  Port=3
  roll_angle_T : Inport  Port=4
  dEFF : Inport  Port=5
  CtrlSurfaces[a] : Inport  Port=6
  Bus Creator : BusCreator  Inputs=3
  Compute CX_a : Subsystem
  Compute CY_a : Subsystem
  Compute CZ_a : Subsystem
  Aero-F-Coeffs_a : Outport
  wires:
  Bus Creator/1 -> Aero-F-Coeffs_a/1
  Compute CZ_a/1(CZ_a) -> Bus Creator/3  "CZ_a"
  Compute CY_a/1(CY_a) -> Bus Creator/2  "CY_a"
  Compute CX_a/1(CX_a) -> Bus Creator/1  "CX_a"
  CtrlSurfaces[a]/1 -> Compute CZ_a/4(CtrlSurfaces[a]), Compute CY_a/4(CtrlSurfaces[a])
  roll_angle_T/1 -> Compute CY_a/3(roll_angle_T), Compute CZ_a/3(roll_angle_T)
  alpha_T_index/1 -> Compute CY_a/1(alpha_T_index), Compute CZ_a/1(alpha_T_index)
  dEFF/1 -> Compute CX_a/3(dEFF)
  alpha_T/1 -> Compute CX_a/2(alpha_T)
  Mach_Number_index/1 -> Compute CX_a/1(Mach_Number_index), Compute CY_a/2(Mach_Number_index), Compute CZ_a/2(Mach_Number_index)

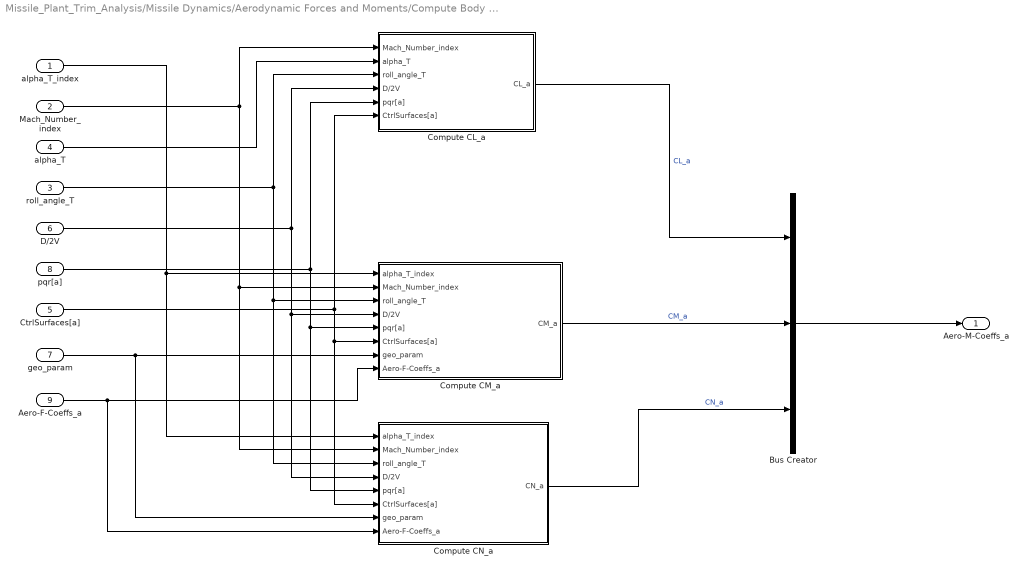
== system Missile_Plant_Trim_Analysis/Missile Dynamics/Aerodynamic Forces and Moments/Compute Body Frame Aerodynamic Forces and Moments/Compute Aeroballistics Frame Aerodynamics Coefficients/Compute Aero-M-Coeffs_a ==
  alpha_T_index : Inport
  Mach_Number_index : Inport  Port=2
  roll_angle_T : Inport  Port=3
  alpha_T : Inport  Port=4
  CtrlSurfaces[a] : Inport  Port=5
  D/2V : Inport  Port=6
  geo_param : Inport  Port=7
  pqr[a] : Inport  Port=8
  Aero-F-Coeffs_a : Inport  Port=9
  Bus Creator : BusCreator  Inputs=3
  Compute CL_a : Subsystem
  Compute CM_a : Subsystem
  Compute CN_a : Subsystem
  Aero-M-Coeffs_a : Outport
  wires:
  Compute CN_a/1(CN_a) -> Bus Creator/3  "CN_a"
  Compute CM_a/1(CM_a) -> Bus Creator/2  "CM_a"
  Aero-F-Coeffs_a/1 -> Compute CN_a/8(Aero-F-Coeffs_a), Compute CM_a/8(Aero-F-Coeffs_a)
  alpha_T_index/1 -> Compute CN_a/1(alpha_T_index), Compute CM_a/1(alpha_T_index)
  geo_param/1 -> Compute CN_a/7(geo_param), Compute CM_a/7(geo_param)
  Compute CL_a/1(CL_a) -> Bus Creator/1  "CL_a"
  CtrlSurfaces[a]/1 -> Compute CL_a/6(CtrlSurfaces[a]), Compute CN_a/6(CtrlSurfaces[a]), Compute CM_a/6(CtrlSurfaces[a])
  pqr[a]/1 -> Compute CL_a/5(pqr[a]), Compute CN_a/5(pqr[a]), Compute CM_a/5(pqr[a])
  D/2V/1 -> Compute CL_a/4(D/2V), Compute CN_a/4(D/2V), Compute CM_a/4(D/2V)
  roll_angle_T/1 -> Compute CL_a/3(roll_angle_T), Compute CN_a/3(roll_angle_T), Compute CM_a/3(roll_angle_T)
  alpha_T/1 -> Compute CL_a/2(alpha_T)
  Mach_Number_index/1 -> Compute CL_a/1(Mach_Number_index), Compute CN_a/2(Mach_Number_index), Compute CM_a/2(Mach_Number_index)
  Bus Creator/1 -> Aero-M-Coeffs_a/1

== system Missile_Plant_Trim_Analysis/Missile Dynamics/Aerodynamic Forces and Moments/Compute Body Frame Aerodynamic Forces and Moments/Compute Aeroballistics Frame Aerodynamics Coefficients/Calculate Coefficient Parameters/Calculate D//2V ==
  <air_speed> : Inport
  D : Inport  Port=2
  Divide : Product  Inputs=*/
  Gain : Gain  Gain=2
  D/2V : Outport
  wires:
  D/1 -> Divide/1
  <air_speed>/1 -> Gain/1
  Divide/1 -> D/2V/1
  Gain/1 -> Divide/2

== system Missile_Plant_Trim_Analysis/Missile Dynamics/Aerodynamic Forces and Moments/Compute Body Frame Aerodynamic Forces and Moments/Compute Aeroballistics Frame Aerodynamics Coefficients/Calculate Coefficient Parameters/Calculate Effective Control Input ==
  <dP> : Inport
  <dY> : Inport  Port=2
  Abs : Abs
  Abs1 : Abs
  Constant : Constant  Value=2
  Divide : Product  Inputs=*/
  Plus : Sum
  dEFF : Outport
  wires:
  <dY>/1 -> Abs1/1
  <dP>/1 -> Abs/1
  Divide/1 -> dEFF/1
  Plus/1 -> Divide/1
  Abs/1 -> Plus/1
  Abs1/1 -> Plus/2
  Constant/1 -> Divide/2

== system Missile_Plant_Trim_Analysis/Missile Dynamics/Aerodynamic Forces and Moments/Compute Body Frame Aerodynamic Forces and Moments/Compute Aeroballistics Frame Aerodynamics Coefficients/Calculate Coefficient Parameters/Calculate Total Angle-of-Attack ==
  <alpha> : Inport
  <beta> : Inport  Port=2
  Acos : Trigonometry  Operator=acos
  Cos : Trigonometry  Operator=cos
  Cos1 : Trigonometry  Operator=cos
  Display : Display
  Product : Product
  alpha_T : Outport
  wires:
  <alpha>/1 -> Cos/1
  Cos1/1 -> Product/2
  Product/1 -> Acos/1
  Acos/1 -> Display/1, alpha_T/1
  Cos/1 -> Product/1
  <beta>/1 -> Cos1/1

== system Missile_Plant_Trim_Analysis/Missile Dynamics/Aerodynamic Forces and Moments/Compute Body Frame Aerodynamic Forces and Moments/Compute Aeroballistics Frame Aerodynamics Coefficients/Calculate Coefficient Parameters/Calculate Total Roll Angle ==
  <alpha> : Inport
  <beta> : Inport  Port=2
  Atan2 : Trigonometry  Operator=atan2
  Sin : Trigonometry
  Tan : Trigonometry  Operator=tan
  roll_angle_T : Outport
  wires:
  Atan2/1 -> roll_angle_T/1
  <alpha>/1 -> Sin/1
  Sin/1 -> Atan2/2  "sin(alpha)"
  <beta>/1 -> Tan/1
  Tan/1 -> Atan2/1  "tan(beta)"

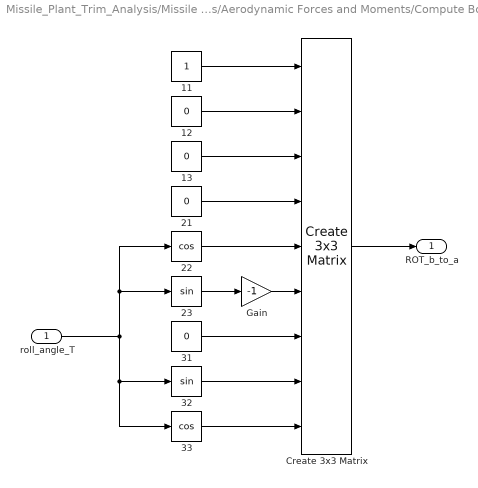
== system Missile_Plant_Trim_Analysis/Missile Dynamics/Aerodynamic Forces and Moments/Compute Body Frame Aerodynamic Forces and Moments/Compute Aeroballistics Frame Aerodynamics Coefficients/Calculate Coefficient Parameters/Compose ROT_b_to_a ==
  roll_angle_T : Inport
  11 : Constant
  {12..13,21,31} (4 alike) : Constant  Value=0
  22 : Trigonometry  Operator=cos
  23 : Trigonometry
  32 : Trigonometry
  33 : Trigonometry  Operator=cos
  Create 3x3 Matrix : sharedutil/Create 3x3 Matrix  aMode=aMode
      settings: SourceProductBaseCode=AE,PW,DR,MT,UV,VE
  Gain : Gain  Gain=-1
  ROT_b_to_a : Outport
  wires:
  Create 3x3 Matrix/1 -> ROT_b_to_a/1
  33/1 -> Create 3x3 Matrix/9
  32/1 -> Create 3x3 Matrix/8
  31/1 -> Create 3x3 Matrix/7
  Gain/1 -> Create 3x3 Matrix/6
  22/1 -> Create 3x3 Matrix/5
  21/1 -> Create 3x3 Matrix/4
  13/1 -> Create 3x3 Matrix/3
  12/1 -> Create 3x3 Matrix/2
  11/1 -> Create 3x3 Matrix/1
  23/1 -> Gain/1
  roll_angle_T/1 -> 22/1, 23/1, 32/1, 33/1

== system Missile_Plant_Trim_Analysis/Missile Dynamics/Aerodynamic Forces and Moments/Compute Body Frame Aerodynamic Forces and Moments/Compute Aeroballistics Frame Aerodynamics Coefficients/Calculate Coefficient Parameters/Convert CtrlSurfaces[b] to CtrlSurfaces[b][a] ==
  ROT_b_to_a : Inport
  CtrlSurfaces[b] : Inport  Port=2
  Matrix Multiply : Product  Multiplication=Matrix(*)
  CtrlSurfaces[a] : Outport
  wires:
  CtrlSurfaces[b]/1 -> Matrix Multiply/2
  ROT_b_to_a/1 -> Matrix Multiply/1
  Matrix Multiply/1 -> CtrlSurfaces[a]/1

== system Missile_Plant_Trim_Analysis/Missile Dynamics/Aerodynamic Forces and Moments/Compute Body Frame Aerodynamic Forces and Moments/Compute Aeroballistics Frame Aerodynamics Coefficients/Calculate Coefficient Parameters/Convert pqr[b] to pqr[a] ==
  ROT_b_to_a : Inport
  pqr[b] : Inport  Port=2
  Matrix Multiply : Product  Multiplication=Matrix(*)
  pqr[a] : Outport
  wires:
  pqr[b]/1 -> Matrix Multiply/2
  ROT_b_to_a/1 -> Matrix Multiply/1
  Matrix Multiply/1 -> pqr[a]/1

== system Missile_Plant_Trim_Analysis/Missile Dynamics/Aerodynamic Forces and Moments/Compute Body Frame Aerodynamic Forces and Moments/Compute Aeroballistics Frame Aerodynamics Coefficients/Calculate Coefficient Parameters/Subsystem ==
  D : Inport
  Divide : Product  Inputs=*/
  Minus : Sum  Inputs=+-
  Missile C.G. Point : Constant  Value=XCG
  Missile Moment Reference Point : Constant  Value=XREF
  geo_param : Outport
  wires:
  Minus/1 -> Divide/1
  Divide/1 -> geo_param/1
  D/1 -> Divide/2
  Missile Moment Reference Point/1 -> Minus/2
  Missile C.G. Point/1 -> Minus/1

== system Missile_Plant_Trim_Analysis/Missile Dynamics/Aerodynamic Forces and Moments/Compute Body Frame Aerodynamic Forces and Moments/Compute Aeroballistics Frame Aerodynamics Coefficients/Compute Aero-F-Coeffs_a/Compute CX_a ==
  Mach_Number_index : Inport
  alpha_T : Inport  Port=2
  dEFF : Inport  Port=3
  Add : Sum  Inputs=+++
  Bus Selector : BusSelector  OutputSignals=k,f
  CX_0 : Interpolation_n-D  NumberOfTableDimensions=1  Table=Tbl_CX_0  InternalRulePriority=Speed
      settings: InputPortMap=u0,u1
  CX_ALPHAT : Interpolation_n-D  NumberOfTableDimensions=1  Table=Tbl_CX_ALPHAT  InternalRulePriority=Speed
      settings: InputPortMap=u0,u1
  CX_DEL_EFF : Interpolation_n-D  NumberOfTableDimensions=1  Table=Tbl_CX_DEL_EFF  InternalRulePriority=Speed
      settings: InputPortMap=u0,u1
  Math Function : Math  Operator=square  SaturateOnIntegerOverflow=on
  Product : Product
  Product1 : Product
  CX_a : Outport
  wires:
  Add/1 -> CX_a/1
  Product1/1 -> Add/3
  Product/1 -> Add/2
  CX_0/1 -> Add/1
  Math Function/1 -> Product1/2
  CX_DEL_EFF/1 -> Product1/1
  dEFF/1 -> Math Function/1
  alpha_T/1 -> Product/2
  CX_ALPHAT/1 -> Product/1
  Bus Selector/2 -> CX_0/2, CX_ALPHAT/2, CX_DEL_EFF/2  "<f>"
  Bus Selector/1 -> CX_0/1, CX_ALPHAT/1, CX_DEL_EFF/1  "<k>"
  Mach_Number_index/1 -> Bus Selector/1

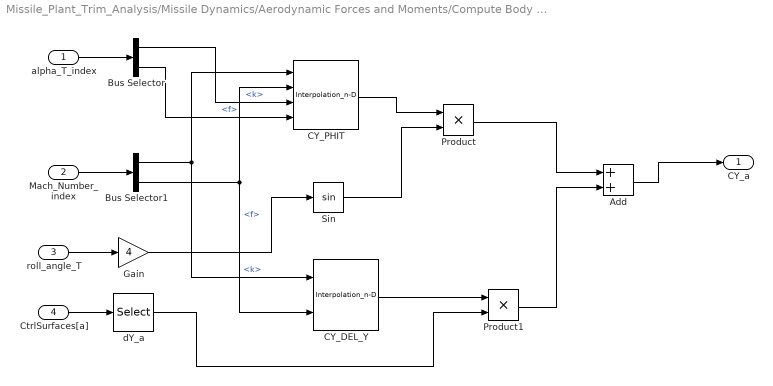
== system Missile_Plant_Trim_Analysis/Missile Dynamics/Aerodynamic Forces and Moments/Compute Body Frame Aerodynamic Forces and Moments/Compute Aeroballistics Frame Aerodynamics Coefficients/Compute Aero-F-Coeffs_a/Compute CY_a ==
  alpha_T_index : Inport
  Mach_Number_index : Inport  Port=2
  roll_angle_T : Inport  Port=3
  CtrlSurfaces[a] : Inport  Port=4
  Add : Sum
  Bus Selector : BusSelector  OutputSignals=k,f
  Bus Selector1 : BusSelector  OutputSignals=k,f
  CY_DEL_Y : Interpolation_n-D  NumberOfTableDimensions=1  Table=Tbl_CY_DEL_Y  InternalRulePriority=Speed
      settings: InputPortMap=u0,u1
  CY_PHIT : Interpolation_n-D  Table=Tbl_CY_PHIT  InternalRulePriority=Speed
  Gain : Gain  Gain=4
  Product : Product
  Product1 : Product
  Sin : Trigonometry
  dY_a : Selector  InputPortWidth=3  IndexOptions=Index vector (dialog)  Indices=[3]  OutputSizes=1
  CY_a : Outport
  wires:
  Bus Selector/2 -> CY_PHIT/4  "<f>"
  Bus Selector/1 -> CY_PHIT/3  "<k>"
  Add/1 -> CY_a/1
  Product1/1 -> Add/2
  dY_a/1 -> Product1/2
  CY_DEL_Y/1 -> Product1/1
  Product/1 -> Add/1
  Sin/1 -> Product/2
  Gain/1 -> Sin/1
  roll_angle_T/1 -> Gain/1
  CY_PHIT/1 -> Product/1
  Bus Selector1/2 -> CY_DEL_Y/2, CY_PHIT/2  "<f>"
  Bus Selector1/1 -> CY_DEL_Y/1, CY_PHIT/1  "<k>"
  CtrlSurfaces[a]/1 -> dY_a/1
  Mach_Number_index/1 -> Bus Selector1/1
  alpha_T_index/1 -> Bus Selector/1

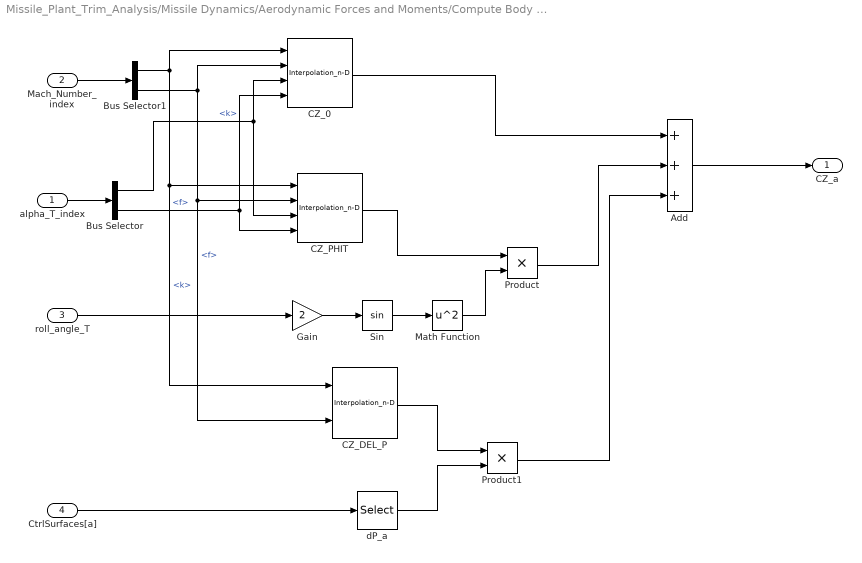
== system Missile_Plant_Trim_Analysis/Missile Dynamics/Aerodynamic Forces and Moments/Compute Body Frame Aerodynamic Forces and Moments/Compute Aeroballistics Frame Aerodynamics Coefficients/Compute Aero-F-Coeffs_a/Compute CZ_a ==
  alpha_T_index : Inport
  Mach_Number_index : Inport  Port=2
  roll_angle_T : Inport  Port=3
  CtrlSurfaces[a] : Inport  Port=4
  Add : Sum  Inputs=+++
  Bus Selector : BusSelector  OutputSignals=k,f
  Bus Selector1 : BusSelector  OutputSignals=k,f
  CZ_0 : Interpolation_n-D  Table=Tbl_CZ_0  InternalRulePriority=Speed
  CZ_DEL_P : Interpolation_n-D  NumberOfTableDimensions=1  Table=Tbl_CZ_DEL_P  InternalRulePriority=Speed
      settings: InputPortMap=u0,u1
  CZ_PHIT : Interpolation_n-D  Table=Tbl_CZ_PHIT  InternalRulePriority=Speed
  Gain : Gain  Gain=2
  Math Function : Math  Operator=square  SaturateOnIntegerOverflow=on
  Product : Product
  Product1 : Product
  Sin : Trigonometry
  dP_a : Selector  InputPortWidth=3  IndexOptions=Index vector (dialog)  Indices=[2]  OutputSizes=1
  CZ_a : Outport
  wires:
  Bus Selector/2 -> CZ_0/4, CZ_PHIT/4  "<f>"
  Bus Selector/1 -> CZ_0/3, CZ_PHIT/3  "<k>"
  Add/1 -> CZ_a/1
  Product1/1 -> Add/3
  Product/1 -> Add/2
  CZ_0/1 -> Add/1
  dP_a/1 -> Product1/2
  CZ_DEL_P/1 -> Product1/1
  Math Function/1 -> Product/2
  CZ_PHIT/1 -> Product/1
  Sin/1 -> Math Function/1
  Gain/1 -> Sin/1
  roll_angle_T/1 -> Gain/1
  Bus Selector1/2 -> CZ_0/2, CZ_PHIT/2, CZ_DEL_P/2  "<f>"
  Bus Selector1/1 -> CZ_0/1, CZ_PHIT/1, CZ_DEL_P/1  "<k>"
  CtrlSurfaces[a]/1 -> dP_a/1
  Mach_Number_index/1 -> Bus Selector1/1
  alpha_T_index/1 -> Bus Selector/1

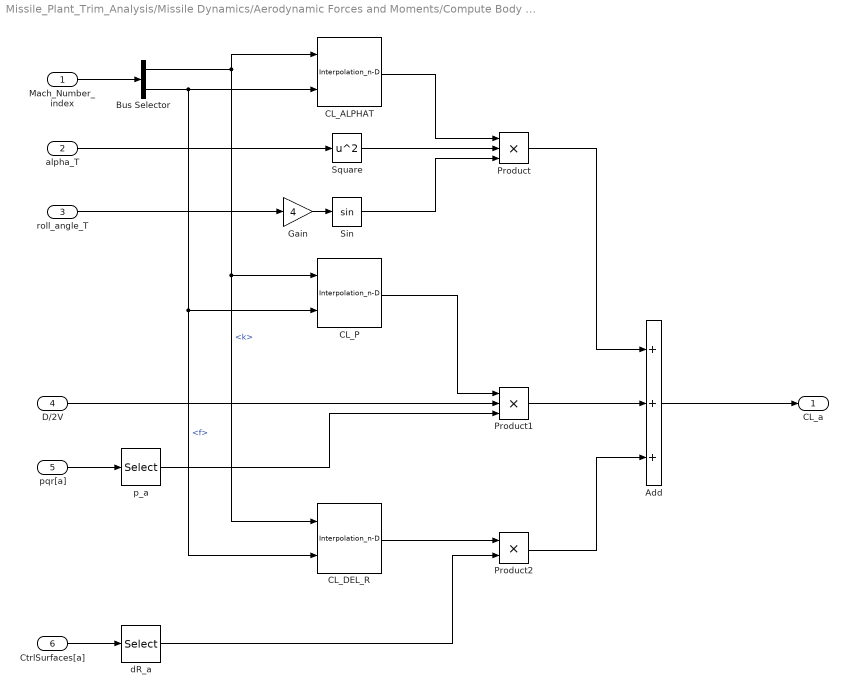
== system Missile_Plant_Trim_Analysis/Missile Dynamics/Aerodynamic Forces and Moments/Compute Body Frame Aerodynamic Forces and Moments/Compute Aeroballistics Frame Aerodynamics Coefficients/Compute Aero-M-Coeffs_a/Compute CL_a ==
  Mach_Number_index : Inport
  alpha_T : Inport  Port=2
  roll_angle_T : Inport  Port=3
  D/2V : Inport  Port=4
  pqr[a] : Inport  Port=5
  CtrlSurfaces[a] : Inport  Port=6
  Add : Sum  Inputs=+++
  Bus Selector : BusSelector  OutputSignals=k,f
  CL_ALPHAT : Interpolation_n-D  NumberOfTableDimensions=1  Table=Tbl_CL_ALPHAT  InternalRulePriority=Speed
      settings: InputPortMap=u0,u1
  CL_DEL_R : Interpolation_n-D  NumberOfTableDimensions=1  Table=Tbl_CL_DEL_R  InternalRulePriority=Speed
      settings: InputPortMap=u0,u1
  CL_P : Interpolation_n-D  NumberOfTableDimensions=1  Table=Tbl_CL_P  InternalRulePriority=Speed
      settings: InputPortMap=u0,u1
  Gain : Gain  Gain=4
  Product : Product  Inputs=3
  Product1 : Product  Inputs=3
  Product2 : Product
  Sin : Trigonometry
  Square : Math  Operator=square  SaturateOnIntegerOverflow=on
  dR_a : Selector  InputPortWidth=3  IndexOptions=Index vector (dialog)  Indices=[1]  OutputSizes=1
  p_a : Selector  InputPortWidth=3  IndexOptions=Index vector (dialog)  Indices=[1]  OutputSizes=1
  CL_a : Outport
  wires:
  Add/1 -> CL_a/1
  Product2/1 -> Add/3
  Product1/1 -> Add/2
  Product/1 -> Add/1
  dR_a/1 -> Product2/2
  CL_DEL_R/1 -> Product2/1
  CtrlSurfaces[a]/1 -> dR_a/1
  p_a/1 -> Product1/3
  D/2V/1 -> Product1/2
  CL_P/1 -> Product1/1
  pqr[a]/1 -> p_a/1
  Sin/1 -> Product/3
  Square/1 -> Product/2
  CL_ALPHAT/1 -> Product/1
  Gain/1 -> Sin/1
  roll_angle_T/1 -> Gain/1
  alpha_T/1 -> Square/1
  Bus Selector/2 -> CL_ALPHAT/2, CL_P/2, CL_DEL_R/2  "<f>"
  Bus Selector/1 -> CL_ALPHAT/1, CL_P/1, CL_DEL_R/1  "<k>"
  Mach_Number_index/1 -> Bus Selector/1

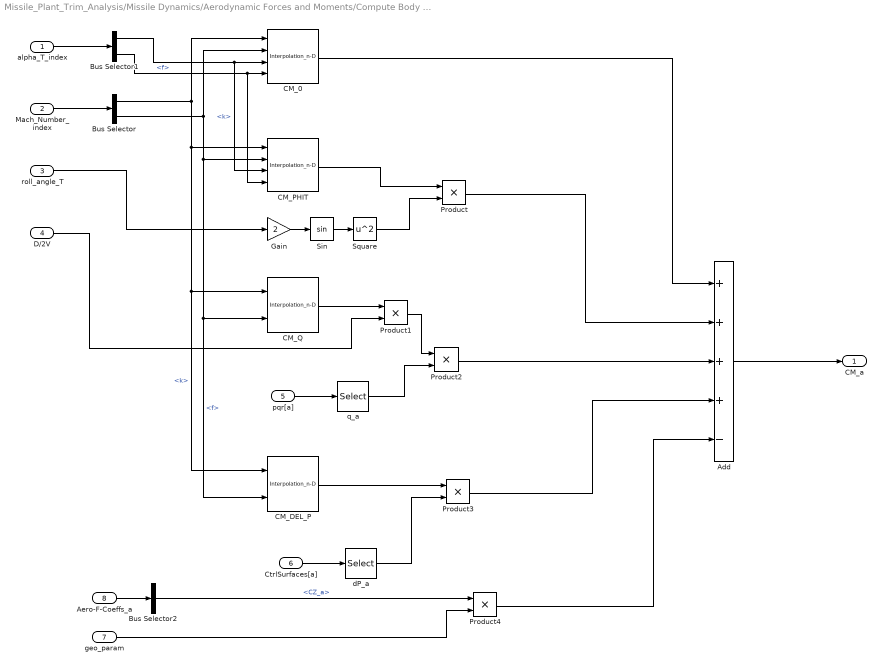
== system Missile_Plant_Trim_Analysis/Missile Dynamics/Aerodynamic Forces and Moments/Compute Body Frame Aerodynamic Forces and Moments/Compute Aeroballistics Frame Aerodynamics Coefficients/Compute Aero-M-Coeffs_a/Compute CM_a ==
  alpha_T_index : Inport
  Mach_Number_index : Inport  Port=2
  roll_angle_T : Inport  Port=3
  D/2V : Inport  Port=4
  pqr[a] : Inport  Port=5
  CtrlSurfaces[a] : Inport  Port=6
  geo_param : Inport  Port=7
  Aero-F-Coeffs_a : Inport  Port=8
  Add : Sum  Inputs=++++-
  Bus Selector : BusSelector  OutputSignals=k,f
  Bus Selector1 : BusSelector  OutputSignals=k,f
  Bus Selector2 : BusSelector  OutputSignals=CZ_a
  CM_0 : Interpolation_n-D  Table=Tbl_CM_0  InternalRulePriority=Speed
  CM_DEL_P : Interpolation_n-D  NumberOfTableDimensions=1  Table=Tbl_CM_DEL_P  InternalRulePriority=Speed
      settings: InputPortMap=u0,u1
  CM_PHIT : Interpolation_n-D  Table=Tbl_CM_PHIT  InternalRulePriority=Speed
  CM_Q : Interpolation_n-D  NumberOfTableDimensions=1  Table=Tbl_CM_Q  InternalRulePriority=Speed
      settings: InputPortMap=u0,u1
  Gain : Gain  Gain=2
  Product{,1..4} (5 alike) : Product
  Sin : Trigonometry
  Square : Math  Operator=square  SaturateOnIntegerOverflow=on
  dP_a : Selector  InputPortWidth=3  IndexOptions=Index vector (dialog)  Indices=[2]  OutputSizes=1
  q_a : Selector  InputPortWidth=3  IndexOptions=Index vector (dialog)  Indices=[2]  OutputSizes=1
  CM_a : Outport
  wires:
  Bus Selector1/2 -> CM_PHIT/4, CM_0/4  "<f>"
  Bus Selector1/1 -> CM_PHIT/3, CM_0/3  "<k>"
  Add/1 -> CM_a/1
  Product4/1 -> Add/5
  Product3/1 -> Add/4
  Product2/1 -> Add/3
  Product/1 -> Add/2
  CM_0/1 -> Add/1
  geo_param/1 -> Product4/2
  Bus Selector2/1 -> Product4/1  "<CZ_a>"
  Aero-F-Coeffs_a/1 -> Bus Selector2/1
  dP_a/1 -> Product3/2
  CM_DEL_P/1 -> Product3/1
  q_a/1 -> Product2/2
  Product1/1 -> Product2/1
  D/2V/1 -> Product1/2
  CM_Q/1 -> Product1/1
  Square/1 -> Product/2
  CM_PHIT/1 -> Product/1
  Sin/1 -> Square/1
  Gain/1 -> Sin/1
  roll_angle_T/1 -> Gain/1
  Bus Selector/2 -> CM_0/2, CM_PHIT/2, CM_DEL_P/2, CM_Q/2  "<f>"
  Bus Selector/1 -> CM_0/1, CM_PHIT/1, CM_Q/1, CM_DEL_P/1  "<k>"
  alpha_T_index/1 -> Bus Selector1/1
  CtrlSurfaces[a]/1 -> dP_a/1
  pqr[a]/1 -> q_a/1
  Mach_Number_index/1 -> Bus Selector/1

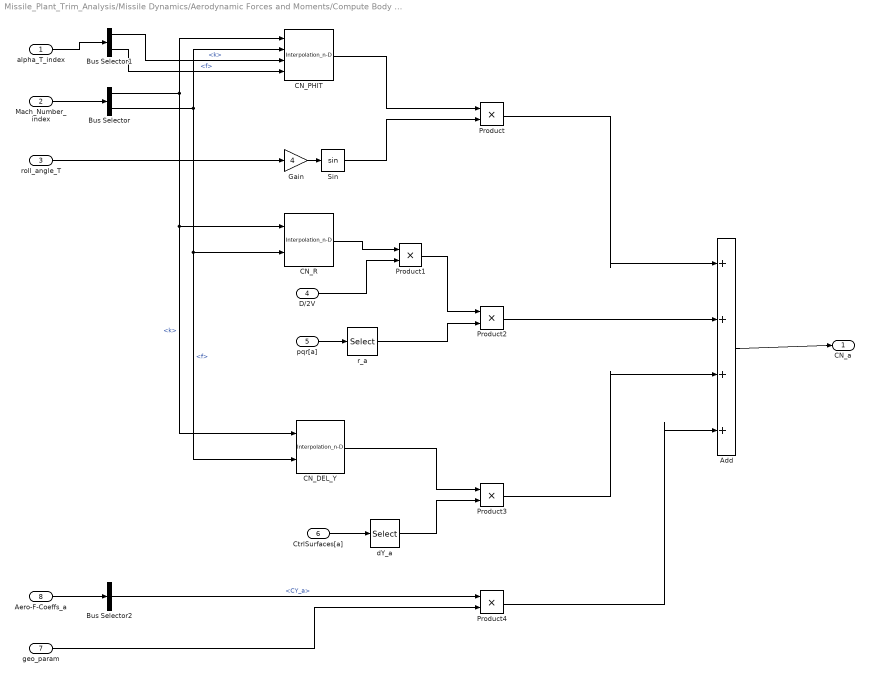
== system Missile_Plant_Trim_Analysis/Missile Dynamics/Aerodynamic Forces and Moments/Compute Body Frame Aerodynamic Forces and Moments/Compute Aeroballistics Frame Aerodynamics Coefficients/Compute Aero-M-Coeffs_a/Compute CN_a ==
  alpha_T_index : Inport
  Mach_Number_index : Inport  Port=2
  roll_angle_T : Inport  Port=3
  D/2V : Inport  Port=4
  pqr[a] : Inport  Port=5
  CtrlSurfaces[a] : Inport  Port=6
  geo_param : Inport  Port=7
  Aero-F-Coeffs_a : Inport  Port=8
  Add : Sum  Inputs=++++
  Bus Selector : BusSelector  OutputSignals=k,f
  Bus Selector1 : BusSelector  OutputSignals=k,f
  Bus Selector2 : BusSelector  OutputSignals=CY_a
  CN_DEL_Y : Interpolation_n-D  NumberOfTableDimensions=1  Table=Tbl_CN_DEL_Y  InternalRulePriority=Speed
      settings: InputPortMap=u0,u1
  CN_PHIT : Interpolation_n-D  Table=Tbl_CN_PHIT  InternalRulePriority=Speed
  CN_R : Interpolation_n-D  NumberOfTableDimensions=1  Table=Tbl_CN_R  InternalRulePriority=Speed
      settings: InputPortMap=u0,u1
  Gain : Gain  Gain=4
  Product{,1..4} (5 alike) : Product
  Sin : Trigonometry
  dY_a : Selector  InputPortWidth=3  IndexOptions=Index vector (dialog)  Indices=[3]  OutputSizes=1
  r_a : Selector  InputPortWidth=3  IndexOptions=Index vector (dialog)  Indices=[3]  OutputSizes=1
  CN_a : Outport
  wires:
  Bus Selector1/2 -> CN_PHIT/4  "<f>"
  Bus Selector1/1 -> CN_PHIT/3  "<k>"
  Add/1 -> CN_a/1
  Product4/1 -> Add/4
  Product3/1 -> Add/3
  Product2/1 -> Add/2
  Product/1 -> Add/1
  geo_param/1 -> Product4/2
  Bus Selector2/1 -> Product4/1  "<CY_a>"
  dY_a/1 -> Product3/2
  CN_DEL_Y/1 -> Product3/1
  CtrlSurfaces[a]/1 -> dY_a/1
  r_a/1 -> Product2/2
  Product1/1 -> Product2/1
  pqr[a]/1 -> r_a/1
  D/2V/1 -> Product1/2
  CN_R/1 -> Product1/1
  Sin/1 -> Product/2
  CN_PHIT/1 -> Product/1
  Gain/1 -> Sin/1
  roll_angle_T/1 -> Gain/1
  Bus Selector/2 -> CN_DEL_Y/2, CN_R/2, CN_PHIT/2  "<f>"
  Bus Selector/1 -> CN_DEL_Y/1, CN_R/1, CN_PHIT/1  "<k>"
  Aero-F-Coeffs_a/1 -> Bus Selector2/1
  alpha_T_index/1 -> Bus Selector1/1
  Mach_Number_index/1 -> Bus Selector/1
